simulink subsystem "Piero"  (R2023b)
settings: Solver=VariableStepAuto  StartTime=0.0  StopTime=10.0  RelTol=1e-3
settings Model: Creator=Usuario  LastModifiedBy=Usuario_UMA

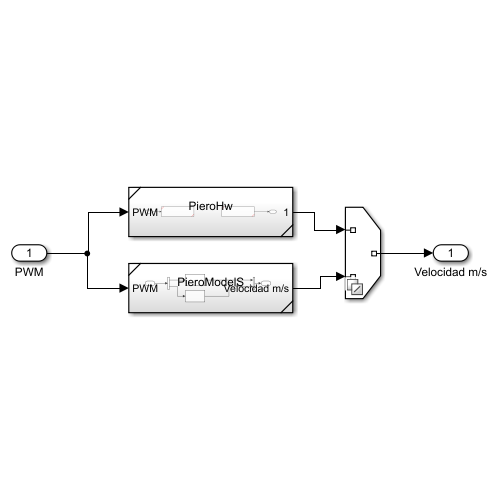
[thumbnail: Simulink's stored preview of the top-level diagram]
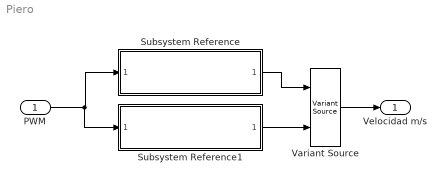
== system Piero ==
  PWM : Inport
  Subsystem Reference : Subsystem  ReferencedSubsystem=PieroHw
  Subsystem Reference1 : Subsystem  ReferencedSubsystem=PieroModelS
  Variant Source : VariantSource  VariantControlMode=sim codegen switching
  Velocidad m/s : Outport
  wires:
  Subsystem Reference1/1 -> Variant Source/2
  PWM/1 -> Subsystem Reference/1, Subsystem Reference1/1
  Variant Source/1 -> Velocidad m/s/1
  Subsystem Reference/1 -> Variant Source/1
